simulink model "Reforce_Experiment_FCS"  (R2021a)
settings: Solver=FixedStepDiscrete  StartTime=0.0  StopTime=Inf  FixedStep=Ts  RelTol=1e-3
PostLoadFcn:
  | , if any(exist('dsrtsu_mdlpostloadfcn', 'file') ~= 0), dsrtsu_mdlpostloadfcn('Execute', bdroot); end,
InitFcn:
  | , if any(exist('rtifpga_mdlclblib', 'file') ~= 0), rtifpga_mdlclblib('Init', bdroot); end,
model workspace (MAT data in the model file):
  FPGA_Control_Scheme_1_Buffer_1_1_1_write = Simulink.Signal
  FPGA_Control_Scheme_1_Buffer_1_1_1_write.Description = 'RTIFPGA'
  FPGA_Control_Scheme_1_Buffer_1_1_1_write.DataType = 'double'
  FPGA_Control_Scheme_1_Buffer_1_1_1_write.Dimensions = '1'
  FPGA_Control_Scheme_1_Buffer_1_1_1_write.DimensionsMode = 'auto'
  FPGA_Control_Scheme_1_Buffer_1_1_1_write.Complexity = 'auto'
  FPGA_Control_Scheme_1_Buffer_1_1_1_write.SampleTime = -1
  FPGA_Control_Scheme_1_Buffer_1_1_1_write.SamplingMode = 'auto'
  FPGA_Control_Scheme_1_Buffer_2_1_1_write = Simulink.Signal
  FPGA_Control_Scheme_1_Buffer_2_1_1_write.Description = 'RTIFPGA'
  FPGA_Control_Scheme_1_Buffer_2_1_1_write.DataType = 'double'
  FPGA_Control_Scheme_1_Buffer_2_1_1_write.Dimensions = '1'
  FPGA_Control_Scheme_1_Buffer_2_1_1_write.DimensionsMode = 'auto'
  FPGA_Control_Scheme_1_Buffer_2_1_1_write.Complexity = 'auto'
  FPGA_Control_Scheme_1_Buffer_2_1_1_write.SampleTime = -1
  FPGA_Control_Scheme_1_Buffer_2_1_1_write.SamplingMode = 'auto'
  FPGA_Control_Scheme_1_Register_1_1_1_write = Simulink.Signal
  FPGA_Control_Scheme_1_Register_1_1_1_write.Description = 'RTIFPGA'
  FPGA_Control_Scheme_1_Register_1_1_1_write.DataType = 'double'
  FPGA_Control_Scheme_1_Register_1_1_1_write.Dimensions = '1'
  FPGA_Control_Scheme_1_Register_1_1_1_write.DimensionsMode = 'auto'
  FPGA_Control_Scheme_1_Register_1_1_1_write.Complexity = 'auto'
  FPGA_Control_Scheme_1_Register_1_1_1_write.SampleTime = -1
  FPGA_Control_Scheme_1_Register_1_1_1_write.SamplingMode = 'auto'
  FPGA_Control_Scheme_1_Register_2_1_1_write = Simulink.Signal
  FPGA_Control_Scheme_1_Register_2_1_1_write.Description = 'RTIFPGA'
  FPGA_Control_Scheme_1_Register_2_1_1_write.DataType = 'double'
  FPGA_Control_Scheme_1_Register_2_1_1_write.Dimensions = '1'
  FPGA_Control_Scheme_1_Register_2_1_1_write.DimensionsMode = 'auto'
  FPGA_Control_Scheme_1_Register_2_1_1_write.Complexity = 'auto'
  FPGA_Control_Scheme_1_Register_2_1_1_write.SampleTime = -1
  FPGA_Control_Scheme_1_Register_2_1_1_write.SamplingMode = 'auto'
values from neighbouring files (symbols this model uses):
  abc2alphabeta0 = [      2/3      -1/3       -1/3 ... (first row only)    [Reforce_Init_FCS.m]
  alphabeta02abc = [  1          0 1/sqrt(2) ... (first row only)    [Reforce_Init_FCS.m]
  torque_ref_sample_lower = -torque_ref_sample_upper    (= -6.5)    [Reforce_Init_FCS.m]
  torque_ref_sample_upper = 6.5    [Reforce_Init_FCS.m]
  Ts = 50e-6    (= 5e-05)    [Reforce_Init_FCS.m]
  uf_factor = U_nom / f_nom    (= 2.82)    [Reforce_Init_FCS.m]
undefined symbols (not defined in the file or in its folder): CC, controller, init_layer_0, init_layer_1, init_layer_2, init_layer_3, init_layer_4, init_layer_5, init_layer_6, init_layer_7, init_layer_8, init_layer_9, inverter, load, motor, PLL, sensor
libraries: simulink x16, rtiproclib x13, rti1202lib_adc_class1 x8, rti1202lib_dio_class1 x4, dspfdesign x3, rtiemclib x2, rti1202lib_dac_class1 x1, embmathops x1, rti1202lib_base x1, rtitasklib x1, dsextras x1, simulink_extras x1
(part 1 of 6)
PostSaveFcn:
  | eval('rtimp_control_gui(''postsave'');', 'disp(lasterr);');
CloseFcn:
  | eval('rtimp_control_gui(''close'');', 'disp(lasterr);');
Description:
  | Standard RTI1202 template.
  | Supported MATLAB version:  R2021a.
settings Model: Tag=RTI1202  DSRTSU_INTERNAL_RTI_VER=580  DSRTSU_INTERNAL_RTI_TYPE=rti1202  RTICANMMDATA=struct('GeneralSetupData',struct('modelroot','C:\Users\Public\RL_Reforce_CCSandFCS','generalsettings',struct('filesettings',struct('destfolder',struct('Name','RTICANMM_FILES','Check',1),'buildfolder',struct('Name','.','Check',1),'AbsDestfolder',struct('Name','C:\Users\Public\RL_Reforce_CCSandFCS\RTICANMM_FILES'),'AbsBuildfolder',struct('Name','C:\Users\Public\RL_Reforce_CCSandFCS'))),'options',struct('addpaths',1,'rmpaths',1,'addtrcexclusion',true,'cannavigator',struct('checkmonitoring',0),'show_usrtrc',0,'use_usrtrc',0),'advanced',struct('options',ones(1,100)),'MPSetup',{{}},'RTI',struct('Type','RTI1202','Ver','7.16','Date','02-May-2021'),'modelname','Reforce_Experiment_FCS','block','Reforce_Experiment_FCS'))  DSRTSU_INTERNAL_RTIFPGA=170  OrderedModelArguments=off  Creator=miro  LastModifiedBy=mschenke
settings SolverCC: AlgebraicLoopSolver=TrustRegion  MinimalZcImpactIntegration=on
settings OptimizationCC: BlockReduction=off  BufferReuse=off  GlobalBufferReuse=off  LocalBlockOutputs=off  EfficientFloat2IntCast=on  SimCompilerOptimization=on  OptimizeDataStoreBuffers=off  BusAssignmentInplaceUpdate=off
settings DebuggingCC: PregeneratedLibrarySubsystemCodeDiagnostic=none  SFMachineParentedDataDiag=warning  ArithmeticOperatorsInVariantConditions=warning
settings HardwareCC: ProdBitPerPointer=32  ProdBitPerSizeT=32  ProdBitPerPtrDiffT=32  ProdLargestAtomicInteger=Integer  ProdEndianess=BigEndian  ProdWordSize=32  ProdLongLongMode=on  ProdHWDeviceType=Custom Processor->Custom  TargetLargestAtomicInteger=Integer  TargetLargestAtomicFloat=Float  TargetLongLongMode=on  TargetIntDivRoundTo=Zero  TargetEndianess=BigEndian  TargetHWDeviceType=Custom Processor->Custom
settings ModelReferenceCC: UpdateModelReferenceTargets=Force  EnableParallelModelReferenceBuilds=on  ParallelModelReferenceMATLABWorkerInit=Load Top Model  ModelReferenceNumInstancesAllowed=Single
settings SFSimCC: SimUseLocalCustomCode=off  MATLABDynamicMemAlloc=off  CustomCodeUndefinedFunction=UseInterfaceOnly  SimHardwareAcceleration=native
settings RTWCC: Description=dSPACE DS1202 Hardware Platform  SystemTargetFile=rti1202.tlc  MakeCommand=make_rti  TemplateMakefile=rti1202.tmf  RTWUseLocalCustomCode=off
settings CodeAppCC: StateflowObjectComments=on
settings STFCustomTargetCC: UtilityFuncGeneration=Shared location  ParMdlRefBuildCompliant=on  GRTInterface=off  UseToolchainInfoCompliant=off  SystemTargetFile=rti1202.tlc
settings GRTTargetCC: TargetLangStandard=C89/C90 (ANSI)  UtilityFuncGeneration=Shared location  CompOptLevelCompliant=off  ConcurrentExecutionCompliant=off  CombineOutputUpdateFcns=off  MatFileLogging=off  CPPClassGenCompliant=off  UseToolchainInfoCompliant=off
settings ConfigComp: CovMetricSettings=dswe

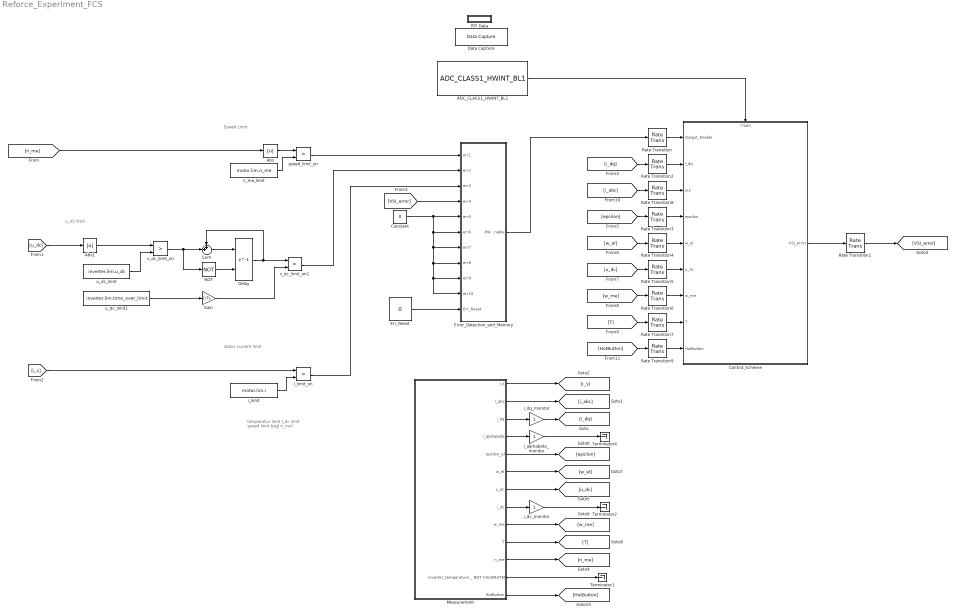
== system Reforce_Experiment_FCS ==
  note: Speed Limit
  note: temperatur limit
      |
      | i_dc limit
      |
      | speed limit bzgl n_me?
  note: u_dc limit
  note: stator current limit
  ADC_CLASS1_HWINT_BL1 : rti1202lib_adc_class1/ADC_CLASS1_HWINT_BL1  DSProperties=struct('RTI',struct('Version',uint32(1),'BlockType',struct('isSLSource',uint8(1),'isSLSink',uint8(0),'isHWSource',uint8(0),'isHWSink',uint8(0),'isSetup',uint8(0),'isInline',uint8(1),'isNonInline',uint8(0),'isInterrupt',uint8(1),'isChannelwise',uint8(0)),'IOBoardType',{{'DS120X','STD','ADCC1'}},'UnitType','DSTASKTOOL','Identifier','HWINT','DialogType','ML','BlockSet','NONE','SlaveProcessor','NONE'))  RTIBlockInterface=struct('OutputPortsActive',1,'OutputPortsWidth',int32(1),'OutputPortsName',{{'Interrupt'}},'FunctionCall',uint32(0),'DialogFcn','rti120xstdadcc1hwintgui','InitLevel',3,'BlockDisplay',{{['ADC CL1 HWINT\nChannel: 1\nInterrupt: Data ready'],'center'}},'IconTransparency','on','BlockName',struct('Token',{{'ADC_CLASS1_HWINT_BL1'}}))  RTIBlockParameters=struct('ChannelNo',{{1,'OFF',[]}},'IntType',{{2,'OFF',[1 3]}})  RTISFcnParameters=struct('ChannelNo','int16','IntType','int16')  RTIBlockParaDefault=struct('ChannelNo',1,'IntType',2)
  Abs : Abs
  Abs1 : Abs
  Constant : Constant  Value=0
  Control_Scheme : Subsystem
  Data Capture : dsextras/Data Capture  ServiceNumber=1  ServiceName=RL_Reforce_Main  SampleTime=-1  XAxisLabelMode=off  XAxisLabel=sec  XAxisIncrement=1  TLCFileName=rti_data_capture  XAxisUnit=[]  IncrementSetting=[]  CustomSampleTime=[]  Reserved1=[]  Reserved2=[]  Reserved3=[]  Reserved4=[]  DSProperties=struct('RTI',struct('Version',uint32(3),'BlockType',struct('isSLSource',uint8(0),'isSLSink',uint8(0),'isHWSource',uint8(0),'isHWSink',uint8(0),'isSetup',uint8(0),'isInline',uint8(1),'isNonInline',uint8(0),'isInterrupt',uint8(0),'isChannelwise',uint8(0)),'IOBoardType','EXTRAS','UnitType','DATACAP','Identifier','DATACAP','DialogType','SL','BlockSet','NONE','SlaveProcessor','NONE'))  RTIBlockInterface=struct('OutputPortsActive',0,'OutputPortsWidth',int32(0),'InitLevel',2,'BlockDisplay',{{['Host Service #1\nRL_Reforce_Main'],'center'}},'BlockName',struct('Token',{{['Data Capture']}}),'MaskDescription',['Places the host service code for ControlDesk in a specific task.'],'IconTransparency','off','SampleTime',{{-1}})  RTIBlockParameters=struct('ServiceNumber',{{1,'OFF',[]}},'ServiceName',{{'RL_Reforce_Main','OFF',[]}},'SampleTime',{{-1,'OFF',[]}},'XAxisLabelMode',{{false,'OFF',[]}},'XAxisLabel',{{'sec','OFF',[]}},'XAxisIncrement',{{1,'OFF',[]}},'TLCFileName',{{'rti_data_capture','OFF',[]}})  RTISFcnParameters=struct('ServiceNumber','double','ServiceName','char','SampleTime','double','XAxisLabelMode','double','XAxisLabel','char','XAxisIncrement','double','TLCFileName','char')  RTIBlockParaDefault=struct('ServiceNumber',1,'ServiceName','<ServiceName>','SampleTime',-1,'XAxisLabelMode',0,'XAxisLabel','sec','XAxisIncrement',1,'TLCFileName','rti_data_capture')
  Delay : Delay  DelayLength=1  ExternalReset=Level  SampleTime=Ts
      settings: InputPortMap=u0,r5
  Err_Reset : Constant  Value=0
  Error_Detection_and_Memory : Subsystem
  Gain : Gain  Gain=1/Ts
  Measurement : Subsystem
  NOT : Logic  Operator=NOT  IconShape=distinctive  AllPortsSameDT=off  OutDataTypeStr=boolean
  RTI Data : Subsystem  Tag=struct('RTIDataServer',struct('RTIDataServerVs','2','RTIModelDescription','struct(''main'',''Reforce_Experiment_FCS'',''sub'','''',''isMp'',0)'))  LoadFcn="if exist('rtidc'), try,  rtidc('DataHostBlockClbLoad', gcbh); catch, disp(['Warning: ''LoadFcn'' for RTI Data block failed: ' lasterr]); end, end,"  mask(RTI_DATA_HOST){}
      mask help:
      | RTI Data Block.
      | This block is used by RTI to store internal model-dependent data.
      | Please keep this block on the root level of the model. Deleting this block will result in data loss.
      |
      | NEVER DELETE OR COPY THIS BLOCK!
      settings: CopyFcn="if exist('rtidc'), try,  rtidc('DataHostBlockClbCopy', gcbh); catch, disp(['Warning: ''CopyFcn'' for RTI Data block failed: ' lasterr]); end, end,"  DeleteFcn="if exist('rtidc'), try,  rtidc('DataHostBlockClbDelete', gcbh); catch, disp(['Warning: ''DeleteFcn'' for RTI Data block failed: ' lasterr]); end, end,"  ModelCloseFcn="if exist('rtidc'), try,  rtidc('DataHostBlockClbModelClose', gcbh); catch, disp(['Warning: ''ModelCloseFcn'' for RTI Data block failed: ' lasterr]); end, end,"  PreSaveFcn="if exist('rtidc'), try,  rtidc('DataHostBlockClbPreSave', gcbh); catch, disp(['Warning: ''PreSaveFcn'' for RTI Data block failed: ' lasterr]); end, end,"  PostSaveFcn="if exist('rtidc'), try,  rtidc('DataHostBlockClbPostSave', gcbh); catch, disp(['Warning: ''PostSaveFcn'' for RTI Data block failed: ' lasterr]); end, end,"  NameChangeFcn="if exist('rtidc'), try,  rtidc('DataHostBlockClbNameChange', gcbh); catch, disp(['Warning: ''NameChangeFcn'' for RTI Data block failed: ' lasterr]); end, end,"
      mask Help:
      | RTI Data Block.
      | This block is used by RTI to store internal model-dependent data.
      | Please keep this block on the root level of the model. Deleting this block will result in data loss.
      | 
      | NEVER DELETE OR COPY THIS BLOCK!
      mask Display:
      | text(0.5, 0.5, 'RTI Data', 'HorizontalAlignment', 'center');
      | plot([1 0]);
  Rate Transition{,1..9} (10 alike) : RateTransition  Deterministic=off
  Sum : Sum  Inputs=++|  AccumDataTypeStr=int32  OutDataTypeStr=int32
  Terminator1 : Terminator
  Terminator2 : Terminator
  Terminator4 : Terminator
  i_alphabeta_monitor : Gain
  i_dc_monitor : Gain
  i_dq_monitor : Gain
  i_limit : Constant  Value=motor.lim.i
  i_limit_on : RelationalOperator  Operator=>  OutDataTypeStr=boolean  RndMeth=Simplest
  n_me_limit : Constant  Value=motor.lim.n_me
  speed_limit_on : RelationalOperator  Operator=>  OutDataTypeStr=boolean  RndMeth=Simplest
  u_dc_limit : Constant  Value=inverter.lim.u_dc
  u_dc_limit1 : Constant  Value=inverter.lim.time_over_limit
  v_dc_limit_on : RelationalOperator  Operator=>  OutDataTypeStr=boolean  RndMeth=Simplest
  v_dc_limit_on1 : RelationalOperator  Operator=>  OutDataTypeStr=boolean  RndMeth=Simplest
  wires:
  ADC_CLASS1_HWINT_BL1/1 -> Control_Scheme/Trigger
  Error_Detection_and_Memory/1(PWM_enable) -> Rate Transition/1
  n_me_limit/1 -> speed_limit_on/2
  Err_Reset/1 -> Error_Detection_and_Memory/11(Err_Reset)
  Rate Transition/1 -> Control_Scheme/1(Output_Enable)
  [n_me] -> Abs/1
  Abs/1 -> speed_limit_on/1
  speed_limit_on/1 -> Error_Detection_and_Memory/1(err1)
  Abs1/1 -> v_dc_limit_on/1
  [u_dc] -> Abs1/1
  u_dc_limit/1 -> v_dc_limit_on/2
  i_limit/1 -> i_limit_on/2
  i_limit_on/1 -> Error_Detection_and_Memory/3(err3)
  Control_Scheme/1(VSI_error) -> Rate Transition1/1
  [i_s] -> i_limit_on/1
  Rate Transition1/1 -> [VSI_error]
  [VSI_error] -> Error_Detection_and_Memory/4(err4)
  Constant/1 -> Error_Detection_and_Memory/10(err10), Error_Detection_and_Memory/9(err9), Error_Detection_and_Memory/8(err8), Error_Detection_and_Memory/7(err7), Error_Detection_and_Memory/6(err6), Error_Detection_and_Memory/5(err5)
  Delay/1 -> v_dc_limit_on1/1, Sum/1
  Sum/1 -> Delay/1
  u_dc_limit1/1 -> Gain/1
  v_dc_limit_on1/1 -> Error_Detection_and_Memory/2(err2)
  NOT/1 -> Delay/2
  Gain/1 -> v_dc_limit_on1/2
  v_dc_limit_on/1 -> NOT/1, Sum/2
  Measurement/3(i_dq) -> i_dq_monitor/1
  Measurement/12(inverter_temperature _ NOT CALIBRATED) -> Terminator1/1
  Measurement/2(i_abc) -> [i_abc]
  i_dq_monitor/1 -> [i_dq]
  Measurement/7(u_dc) -> [u_dc]
  Measurement/1(i_s) -> [i_s]
  Measurement/10(T) -> [T]
  Measurement/4(i_alphabeta) -> i_alphabeta_monitor/1
  Measurement/8(i_dc) -> i_dc_monitor/1
  Measurement/6(w_el) -> [w_el]
  Measurement/9(w_me) -> [w_me]
  Measurement/5(epsilon_el) -> [epsilon]
  Measurement/11(n_me) -> [n_me]
  i_dc_monitor/1 -> Terminator2/1
  i_alphabeta_monitor/1 -> Terminator4/1
  [i_dq] -> Rate Transition2/1
  [epsilon] -> Rate Transition3/1
  [w_el] -> Rate Transition4/1
  [u_dc] -> Rate Transition5/1
  [w_me] -> Rate Transition6/1
  [T] -> Rate Transition7/1
  Rate Transition2/1 -> Control_Scheme/2(i_dq)
  Rate Transition3/1 -> Control_Scheme/4(epsilon)
  Rate Transition4/1 -> Control_Scheme/5(w_el)
  Rate Transition5/1 -> Control_Scheme/6(u_dc)
  Rate Transition6/1 -> Control_Scheme/7(w_me)
  Rate Transition7/1 -> Control_Scheme/8(T)
  Rate Transition8/1 -> Control_Scheme/3(In3)
  [i_abc] -> Rate Transition8/1
  Measurement/13(HotButton) -> [HotButton]
  Rate Transition9/1 -> Control_Scheme/9(HotButton)
  [HotButton] -> Rate Transition9/1
